simulink model "automata_learning"  (R2022a)
settings: Solver=FixedStepAuto  StartTime=0.0  StopTime=10.0  FixedStep=0.005  RelTol=1e-3
settings Model: Creator=diego  LastModifiedBy=diego

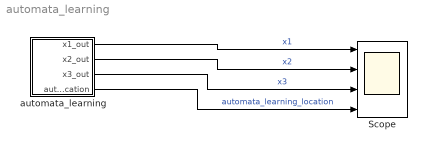
== system automata_learning ==
  Scope : Scope  NumInputPorts=4
  automata_learning : Stateflow chart  TreatAsAtomicUnit=on
  wires:
  automata_learning/1(x1_out) -> Scope/1  "x1"
  automata_learning/2(x2_out) -> Scope/2  "x2"
  automata_learning/3(x3_out) -> Scope/3  "x3"
  automata_learning/4(automata_learning_location) -> Scope/4  "automata_learning_location"

== stateflow chart automata_learning/automata_learning ==
  settings: updateMethod=CONTINUOUS
  state loc1
    du:
    x1_dot = 3.117145091360726 - 6.236726331582759 * x2 - 0.06048766661353966 * x3 - 7.16491395077901 * x1;
    x2_dot = 5.6789874840469565 * x1 + 4.015041317165014 * x2 + 1.472908217470831 * x3 - 5.369614987808745;
    x3_dot = 2.8918727170093916 * x1 + 2.047286249115132 * x2 - 2.2942002437339397 * x3 + 0.3685019598733561;
    x1_out=x1;
    x2_out=x2;
    x3_out=x3;
    automata_learning_location =1;
  state loc2
    du:
    x1_dot = 0.3781958949784894 * x1 + 0.5667232912255713 * x2 + 1.1820176425426325 * x3 + 0.04975323615462912;
    x2_dot = 1.0199052188399946 * x1 - 0.8502210061997175 * x2 + 0.48139552073553205 * x3 + 0.06099497224931838;
    x3_dot = 0.6268806836960721 * x2 - 1.3935050202198909 * x1 - 1.3442249700638058 * x3 - 0.1265419602464135;
    x1_out=x1;
    x2_out=x2;
    x3_out=x3;
    automata_learning_location =2;
  loc1 -> loc2 : [3.613 * x1 + 3.088 * x2 - 2.026 * x3 + 1.0 > 0.0]
  (default) -> loc1 : {x1 = 0.0;
      | x2 = 0.0;
      | x3 = 0.0;}
  data: x1_out output; x1 local; x2_out output; x2 local; x3_out output; x3 local; automata_learning_location output
  data x1 settings: updateMethod=SF_CONTINUOUS_TIME_DATA
  data x2 settings: updateMethod=SF_CONTINUOUS_TIME_DATA
  data x3 settings: updateMethod=SF_CONTINUOUS_TIME_DATA
